simulink model "SystemModel"  (R2017a)
settings: Solver=VariableStepAuto  StartTime=0.0  StopTime=100  RelTol=1e-3
values from neighbouring files (symbols this model uses):
  DroneMomentArm = MomentArm*centi    [System.m]
  ELEC0_DEN = [M0(TermL),M0(TermR)]    [System.m]
  ELEC0_NUM = [1]    [System.m]
  ELEC1_DEN = [M1(TermL),M1(TermR)]    [System.m]
  ELEC1_NUM = [1]    [System.m]
  ELEC2_DEN = [M2(TermL),M2(TermR)]    [System.m]
  ELEC2_NUM = [1]    [System.m]
  ELEC3_DEN = [M3(TermL),M3(TermR)]    [System.m]
  ELEC3_NUM = [1]    [System.m]
  linearizedThrustGain = 0.0027    [System.m]
  M0 = [ ... (first row only)    [MotorSpecs.m]
  M1 = M0    [System.m]
  M2 = M0    [System.m]
  M3 = M0    [System.m]
  MECH0_DEN = [M0(RotJ)+PropellerJ,M0_dyn_fric+linearizedFrictionCoef]    [System.m]
  MECH0_NUM = [1]    [System.m]
  MECH1_DEN = [M1(RotJ)+PropellerJ,M1_dyn_fric+linearizedFrictionCoef]    [System.m]
  MECH1_NUM = [1]    [System.m]
  MECH2_DEN = [M2(RotJ)+PropellerJ,M2_dyn_fric+linearizedFrictionCoef]    [System.m]
  MECH2_NUM = [1]    [System.m]
  MECH3_DEN = [M2(RotJ)+PropellerJ,M3_dyn_fric+linearizedFrictionCoef]    [System.m]
  MECH3_NUM = [1]    [System.m]
  MECHX_D = [DroneJx,0,0]    [System.m]
  MECHX_N = 1    [System.m]
  MECHY_D = [DroneJy,0,0]    [System.m]
  MECHY_N = 1    [System.m]
  SpdK = 12    [Constants.m]
  TorqueK = 11    [Constants.m]
libraries: simulink x3
settings Model: Creator=Matthew  LastModifiedBy=Matthew

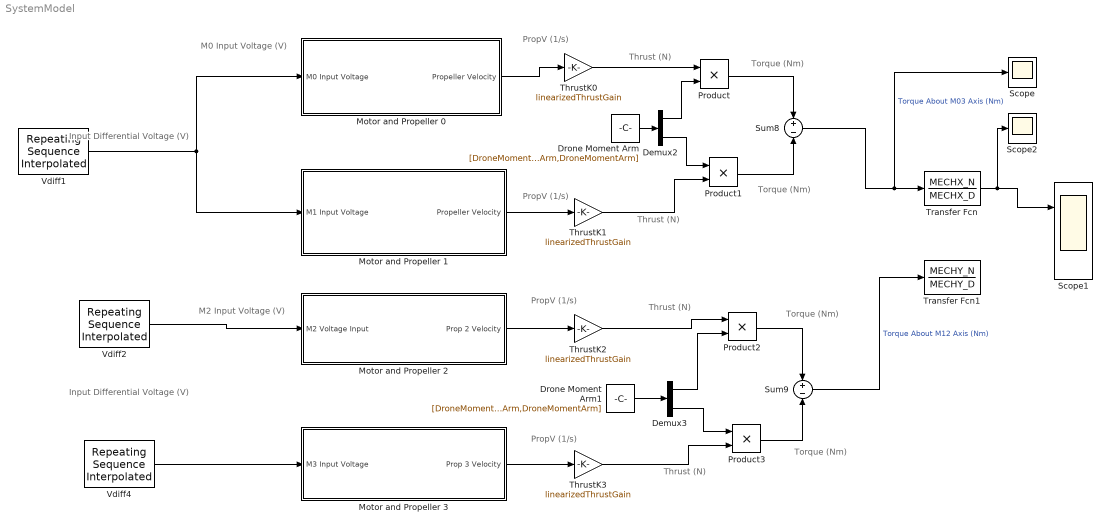
== system SystemModel ==
  note: Torque (Nm)
  note: Thrust (N)
  note: PropV (1/s)
  note: M0 Input Voltage (V)
  note: Input Differential Voltage
      | 		(V)
  note: Input Differential Voltage
      | 		(V)
  note: M2 Input Voltage (V)
  note: PropV (1/s)
  note: PropV (1/s)
  note: PropV (1/s)
  note: Thrust (N)
  note: Thrust (N)
  note: Thrust (N)
  note: Torque (Nm)
  note: Torque (Nm)
  note: Torque (Nm)
  Demux2 : Demux  Outputs=2
  Demux3 : Demux  Outputs=2
  Drone Moment Arm : Constant  Value=[DroneMomentArm,DroneMomentArm]
  Drone Moment Arm1 : Constant  Value=[DroneMomentArm,DroneMomentArm]
  Motor and Propeller 0 : Subsystem
  Motor and Propeller 1 : Subsystem
  Motor and Propeller 2 : Subsystem
  Motor and Propeller 3 : Subsystem
  Product{,1..3} (4 alike) : Product
  Scope : Scope
  Scope1 : Scope  NumInputPorts=2
  Scope2 : Scope
  Sum8 : Sum  Inputs=+|-
  Sum9 : Sum  Inputs=+|-
  "ThrustK0 " : Gain  Gain=linearizedThrustGain
  ThrustK1 : Gain  Gain=linearizedThrustGain
  ThrustK2 : Gain  Gain=linearizedThrustGain
  ThrustK3 : Gain  Gain=linearizedThrustGain
  Transfer Fcn : TransferFcn  Numerator=MECHX_N  Denominator=MECHX_D
  Transfer Fcn1 : TransferFcn  Numerator=MECHY_N  Denominator=MECHY_D
  Vdiff1 : simulink/Sources/Repeating Sequence Interpolated  OutValues=noise_test0  TimeValues=t  LookUpMeth=Use Input Nearest  tsamp=0.01  OutMin=[]  OutMax=[]  OutDataTypeStr=double  OutputDataTypeScalingMode=double  OutDataType=fixdt(0,8)  OutScaling=2^-10
  Vdiff2 : simulink/Sources/Repeating Sequence Interpolated  OutValues=noise_test1  TimeValues=t  LookUpMeth=Interpolation-Use End Values  tsamp=0.01  OutMin=[]  OutMax=[]  OutDataTypeStr=double  OutputDataTypeScalingMode=double  OutDataType=fixdt(0,8)  OutScaling=2^-10
  Vdiff4 : simulink/Sources/Repeating Sequence Interpolated  OutValues=noise_test0  TimeValues=t  LookUpMeth=Interpolation-Use End Values  tsamp=0.01  OutMin=[]  OutMax=[]  OutDataTypeStr=double  OutputDataTypeScalingMode=double  OutDataType=fixdt(0,8)  OutScaling=2^-10
  wires:
  Vdiff2/1 -> Motor and Propeller 2/1(M2 Voltage Input)
  Drone Moment Arm/1 -> Demux2/1
  Drone Moment Arm1/1 -> Demux3/1
  Demux2/1 -> Product/2
  "ThrustK0 "/1 -> Product/1
  Demux2/2 -> Product1/1
  ThrustK1/1 -> Product1/2
  Product/1 -> Sum8/1
  Product1/1 -> Sum8/2
  Product2/1 -> Sum9/1
  Product3/1 -> Sum9/2
  ThrustK2/1 -> Product2/1
  Demux3/1 -> Product2/2
  Demux3/2 -> Product3/1
  ThrustK3/1 -> Product3/2
  Motor and Propeller 0/1(Propeller Velocity) -> "ThrustK0 "/1
  Motor and Propeller 2/1(Prop 2 Velocity) -> ThrustK2/1
  Motor and Propeller 3/1("Prop 3 Velocity ") -> ThrustK3/1
  Motor and Propeller 1/1(Propeller Velocity) -> ThrustK1/1
  Vdiff1/1 -> Motor and Propeller 1/1(M1 Input Voltage), Motor and Propeller 0/1(M0 Input Voltage)
  Vdiff4/1 -> Motor and Propeller 3/1(M3 Input Voltage)
  Sum8/1 -> Scope/1, Transfer Fcn/1  "Torque About M03 Axis \t\t(Nm)"
  Sum9/1 -> Transfer Fcn1/1  "Torque About M12 Axis \t\t(Nm)"
  Transfer Fcn/1 -> Scope2/1, Scope1/1

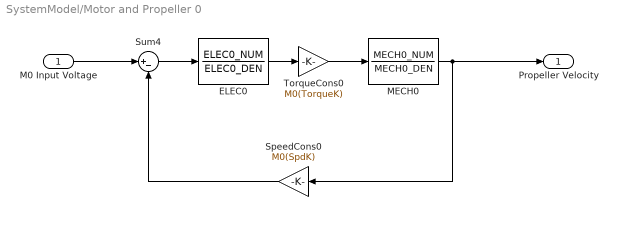
== system SystemModel/Motor and Propeller 0 ==
  M0 Input Voltage : Inport
  ELEC0 : TransferFcn  Numerator=ELEC0_NUM  Denominator=ELEC0_DEN
  MECH0 : TransferFcn  Numerator=MECH0_NUM  Denominator=MECH0_DEN
  SpeedCons0 : Gain  Gain=M0(SpdK)
  Sum4 : Sum  Inputs=|+-
  TorqueCons0 : Gain  Gain=M0(TorqueK)
  Propeller Velocity : Outport
  wires:
  ELEC0/1 -> TorqueCons0/1
  M0 Input Voltage/1 -> Sum4/1
  Sum4/1 -> ELEC0/1
  TorqueCons0/1 -> MECH0/1
  SpeedCons0/1 -> Sum4/2
  MECH0/1 -> Propeller Velocity/1, SpeedCons0/1

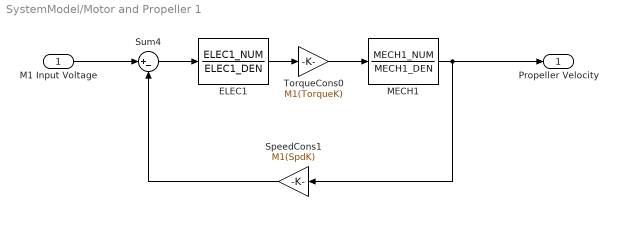
== system SystemModel/Motor and Propeller 1 ==
  M1 Input Voltage : Inport
  ELEC1 : TransferFcn  Numerator=ELEC1_NUM  Denominator=ELEC1_DEN
  MECH1 : TransferFcn  Numerator=MECH1_NUM  Denominator=MECH1_DEN
  SpeedCons1 : Gain  Gain=M1(SpdK)
  Sum4 : Sum  Inputs=|+-
  TorqueCons0 : Gain  Gain=M1(TorqueK)
  Propeller Velocity : Outport
  wires:
  ELEC1/1 -> TorqueCons0/1
  M1 Input Voltage/1 -> Sum4/1
  Sum4/1 -> ELEC1/1
  TorqueCons0/1 -> MECH1/1
  SpeedCons1/1 -> Sum4/2
  MECH1/1 -> Propeller Velocity/1, SpeedCons1/1

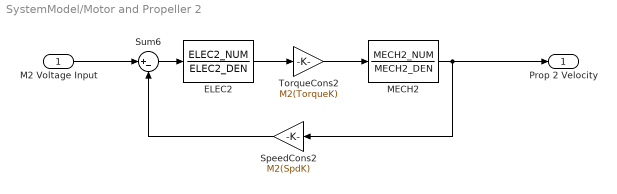
== system SystemModel/Motor and Propeller 2 ==
  M2 Voltage Input : Inport
  ELEC2 : TransferFcn  Numerator=ELEC2_NUM  Denominator=ELEC2_DEN
  MECH2 : TransferFcn  Numerator=MECH2_NUM  Denominator=MECH2_DEN
  SpeedCons2 : Gain  Gain=M2(SpdK)
  Sum6 : Sum  Inputs=|+-
  TorqueCons2 : Gain  Gain=M2(TorqueK)
  Prop 2 Velocity : Outport
  wires:
  Sum6/1 -> ELEC2/1
  ELEC2/1 -> TorqueCons2/1
  MECH2/1 -> Prop 2 Velocity/1, SpeedCons2/1
  TorqueCons2/1 -> MECH2/1
  SpeedCons2/1 -> Sum6/2
  M2 Voltage Input/1 -> Sum6/1

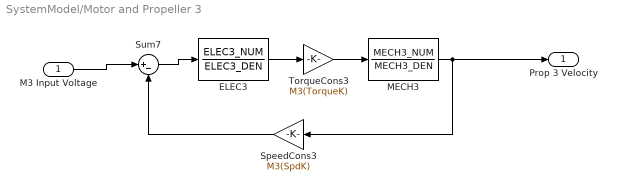
== system SystemModel/Motor and Propeller 3 ==
  M3 Input Voltage : Inport
  ELEC3 : TransferFcn  Numerator=ELEC3_NUM  Denominator=ELEC3_DEN
  MECH3 : TransferFcn  Numerator=MECH3_NUM  Denominator=MECH3_DEN
  SpeedCons3 : Gain  Gain=M3(SpdK)
  Sum7 : Sum  Inputs=|+-
  TorqueCons3 : Gain  Gain=M3(TorqueK)
  "Prop 3 Velocity " : Outport
  wires:
  ELEC3/1 -> TorqueCons3/1
  MECH3/1 -> "Prop 3 Velocity "/1, SpeedCons3/1
  SpeedCons3/1 -> Sum7/2
  TorqueCons3/1 -> MECH3/1
  Sum7/1 -> ELEC3/1
  M3 Input Voltage/1 -> Sum7/1
